simulink model "Modello_Cella_Peltier"  (R2025b)
settings: Solver=ode45  StartTime=0.0  StopTime=6600  FixedStep=0.1  MaxStep=0.5  RelTol=1e-3
libraries: slpidlib x1, simulink x1
settings Model: VariantFading=off  Creator=Lorenzo Raspaolo  LastModifiedBy=Lorenzo Raspaolo
settings SolverCC: ZeroCrossAlgorithm=Adaptive

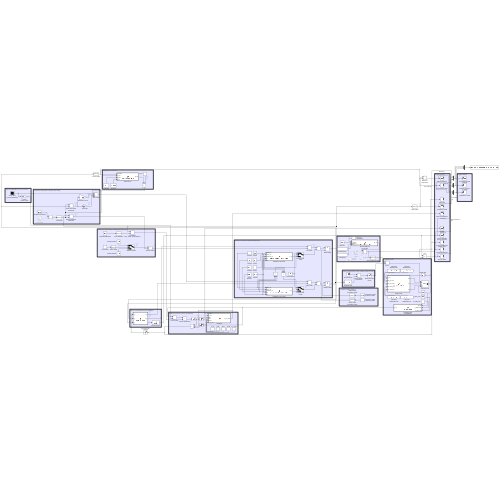
[thumbnail: Simulink's stored preview of the top-level diagram]
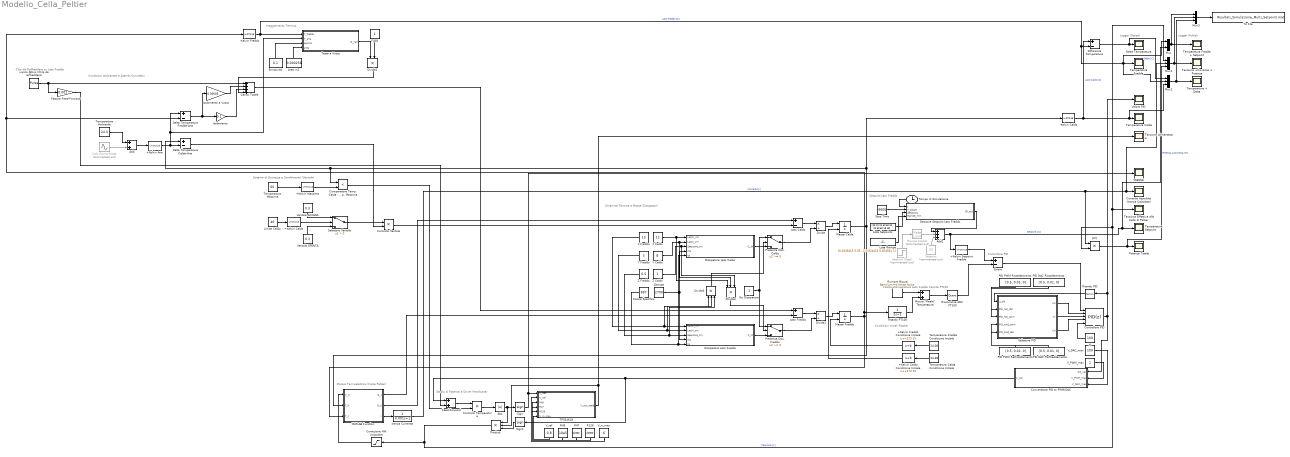
== system Modello_Cella_Peltier ==
  note: Logger Multipli
  note: Condizioni Iniziali Piastre
  note: Sistema di Sicurezza e Smaltimento (Ventola)
  note: Condizioni Ambientali e Scambi Convettivi
  note: Irraggiamento Termico
  note: Dinamica Termica e Masse (Dissipatori)
  note: Motore Termoelettrico (Fisica Peltier)
  note: Stadio di Potenza e Driver (Hardware)
  note: Controllore PID
  note: Logger (Scope)
  note: Calcolo Temperatura Lato Freddo tramite PT100
  note: Setpoint Lato Freddo
  note: Chip da Raffreddare su Lato Freddo
  +Kelvin Aria : Bias  Bias=273.15  SaturateOnIntegerOverflow=off
  +Kelvin Caldo : Bias  Bias=273.15  SaturateOnIntegerOverflow=off
  +Kelvin Caldo Condizione Iniziale : Bias  Bias=+273.15  SaturateOnIntegerOverflow=off
  +Kelvin Freddo Condizione Iniziale : Bias  Bias=+273.15  SaturateOnIntegerOverflow=off
  +Kelvin Massima : Bias  Bias=273.15  SaturateOnIntegerOverflow=off
  +Kelvin Setpoint Freddo : Bias  Bias=273.15  SaturateOnIntegerOverflow=off
  -Kelvin Caldo : Bias  Bias=-273.15  SaturateOnIntegerOverflow=off
  -Kelvin Freddo : Bias  Bias=-273.15  SaturateOnIntegerOverflow=off
  Abs : Abs  SaturateOnIntegerOverflow=off
  Add : Sum
  Add1 : Sum  Inputs=+++
  Area m2 : Constant  Value=0.000256
  Calore Specifico : Constant  Value=897
  Carico Attivo (Chip da raffreddare) : DiscretePulseGenerator  PulseType=Time based  Amplitude=0  Period=36000  PulseWidth=80  PhaseDelay=3600
  Carico Totale : Sum  Inputs=++++
  Ciclo Giorno-Notte : Sin  Commented=on  Bias=25  Frequency=2*pi/36000  SampleTime=0
  Comparatore Temp. Calda - Temp. Massima : RelationalOperator  Operator=<  OutDataTypeStr=boolean  RndMeth=Simplest  InputSameDT=off
  Controllo Temperatura : Product
  Controllo Ventola : Product
  Controllore PID : slpidlib/PID Controller  Controller=PID  Form=Parallel  TimeDomain=Discrete-time  UseExternalTs=off  SampleTime=1  IntegratorMethod=Forward Euler  FilterMethod=Forward Euler  ControllerParametersSource=external  P=1  I=0.7  UseKiTs=off  D=0  UseExternalDerivativeSource=off  N=100  UseFilter=on  TunerSelectOption=Transfer Function Based (PID Tuner App)  InitialConditionSource=internal  InitialConditionForIntegrator=0  InitialConditionForFilter=0  DifferentiatorICPrevScaledInput=0  ExternalReset=none  TrackingMode=off  Kt=1  LimitOutput=on  SatLimitsSource=internal  UpperSaturationLimit=100  LowerSaturationLimit=0  LinearizeAsGain=on  AntiWindupMode=clamping  Kb=1  LimitIntegrator=off  UpperIntegratorSaturationLimit=inf  LowerIntegratorSaturationLimit=-inf  POutMin=[]  POutMax=[]  IOutMin=[]  IOutMax=[]  DOutMin=[]  DOutMax=[]  NOutMin=[]  NOutMax=[]  SumOutMin=[]  SumOutMax=[]  SaturationOutMin=[]  SaturationOutMax=[]  PParamMin=[]  PParamMax=[]  IParamMin=[]  IParamMax=[]  DParamMin=[]  DParamMax=[]  NParamMin=[]  NParamMax=[]  KbParamMin=[]  KbParamMax=[]  KtParamMin=[]  KtParamMax=[]  KbOutMin=[]  KbOutMax=[]  KtOutMin=[]  KtOutMax=[]  IntegratorOutMin=[]  IntegratorOutMax=[]  FilterOutMin=[]  FilterOutMax=[]  SumI1OutMin=[]  SumI1OutMax=[]  SumI2OutMin=[]  SumI2OutMax=[]  SumI3OutMin=[]  SumI3OutMax=[]  SumI4OutMin=[]  SumI4OutMax=[]  SumDOutMin=[]  SumDOutMax=[]  DifferentiatorOutMin=[]  DifferentiatorOutMax=[]  FilterDiffOutCoefMin=[]  FilterDiffOutCoefMax=[]  ReciprocalOutMin=[]  ReciprocalOutMax=[]  SumDenOutMin=[]  SumDenOutMax=[]  SumNumOutMin=[]  SumNumOutMax=[]  DivideOutMin=[]  DivideOutMax=[]  UdiffTsProdOutMin=[]  UdiffTsProdOutMax=[]  NTsProdOutMin=[]  NTsProdOutMax=[]  UintegralTsProdOutMin=[]  UintegralTsProdOutMax=[]  UngainTsProdOutMin=[]  UngainTsProdOutMax=[]  ClampingZeroOutDataTypeStr=Inherit: Inherit via back propagation  ClampingZeroOutMin=[]  ClampingZeroOutMax=[]  FilterDenConstantOutDataTypeStr=Inherit: Inherit via back propagation  FilterDenConstantOutMin=[]  FilterDenConstantOutMax=[]  PCopyOutDataTypeStr=Inherit: Inherit via back propagation  PCopyOutMin=[]  PCopyOutMax=[]  NCopyOutDataTypeStr=Inherit: Inherit via back propagation  NCopyOutMin=[]  NCopyOutMax=[]  IntegratorContinuousStateAttributes=''  IntegratorStateMustResolveToSignalObject=off  IntegratorRTWStateStorageClass=Auto  FilterContinuousStateAttributes=''  FilterStateMustResolveToSignalObject=off  FilterRTWStateStorageClass=Auto  ParallelPVariant=ExternalParameters  IdealPVariant=Disabled  IVariant=ExternalParameters  DVariant=ExternalParameters  IntegratorVariant=Discrete  SatVariant=Enabled  AWVariant=DiscClampingParallel  PCopyVariant=Disabled  TRVariant=Disabled  FdbkBlocksVariant=Forward  IdealPFdbkVariant=Disabled  SatFdbkVariant=Disabled  DerivativeFilterVariant=ForwardEulerFilter  NVariant=ExternalParameters  NCopyVariant=Disabled  FilterICVariant=InternalICsFilter  IntegratorICVariant=InternalICs  ExternalResetVariant=Disabled  TRSumVariant=Passthrough  SumFdbkVariant=Disabled  SumVariant=Sum_PID  TsampFilterVariant=InternalTs  TsampNgainVariant=Passthrough  TsampIntegralVariant=Disabled_SignalSpec  ExternalSaturationOutDataTypeStr=Inherit: Same as second input  DerivativeSourceVariant=ErrorSignal  PreIntVariant=InternalPreInt
  Convertitore PID to PWM/DAC : MATLAB Function  TreatAsAtomicUnit=on
  Corrente Assorbita (Inerzia Calcolata) : Scope
      settings: ActiveDisplayYMinimum=-0.14205533461473169  ActiveDisplayYMaximum=1.2782549500001226  DataLoggingVariableName=ScopeData8
  Correzione HW Unipolare : Saturate  UpperLimit=6  LowerLimit=0
  Decisore Setpoint Lato Freddo : MATLAB Function  TreatAsAtomicUnit=on
  Delta Temperatura : Scope
      settings: ActiveDisplayYMinimum=-1  ActiveDisplayYMaximum=1  DataLoggingVariableName=ScopeData3
  Delta Temperatura Fredda-Aria : Sum  Inputs=+-
  Delta Temperatura Calda-Aria : Sum  Inputs=+-
  Densità : Constant  Value=2700
  Differenza Temperature : Sum  Inputs=+-
  Dissipatore Lato Caldo : MATLAB Function  TreatAsAtomicUnit=on
  Dissipatore Lato Freddo : MATLAB Function  TreatAsAtomicUnit=on
  Divide : Product  Inputs=*/
  Divide1 : Product  Inputs=*/
  Divide2 : Product  Inputs=**
  Divide3 : Product  Inputs=***
  Divide4 : Product  Inputs=***
  Emissività : Constant  Value=0.1
  Errore : Sum  Inputs=+-
  FLAG : Constant
  Fattore Feed-Forward : Gain  Gain=0.001
  Feed-Forward : Sum
  Inerzia Corrente : TransferFcn  Denominator=[0.001, 1]
  Isolamento : Gain  Gain=0.1
  Isolamento a Vuoto : Gain  Gain=0.00005
  Lato Caldo : Sum  Inputs=+-
  Lato Freddo : Sum  Inputs=+-
  Limite Caldo : Constant  Value=40
  Lista Rampe : Constant  Value=[0.0349415 0.0350877 0.298099 0.298246 0.429678 0.429825 0.692836 0.692982 0.824415 0.824561 1]
  Lista Setpoints : Constant  Value=[25 22 22 60 60 20 20 60 60 18 18]
  MATLAB Function : MATLAB Function  TreatAsAtomicUnit=on
  Massa Calda : Integrator  InitialConditionSource=external  InitialCondition=298.15
  Massa Fredda : Integrator  InitialConditionSource=external  InitialCondition=298.15
  "Misura \"Reale\" Temperatura" : Sum
  Mux : Mux  Inputs=2
  Mux1 : Mux  Inputs=3
  Mux2 : Mux  Inputs=3
  Mux3 : Mux  Inputs=3
  N : Constant  Value=100
  No Dissipatore : Constant
  PID DAC Raffreddamento : Constant  Value=[0.5, 0.01, 0]
  PID DAC Riscaldamento : Constant  Value=[0.5, 0.01, 0]
  PID PWM Raffreddamento : Constant  Value=[0.5, 0.01, 0]
  PID PWM Riscaldamento : Constant  Value=[0.5, 0.01, 0]
  Potenza Totale : Scope
      settings: DataLoggingVariableName=ScopeData13
  Presenza Diss. Caldo : Switch  SaturateOnIntegerOverflow=off  InputSameDT=off
  Presenza Diss. Freddo : Switch  SaturateOnIntegerOverflow=off  InputSameDT=off
  Product : Product  Inputs=3
  R126 : Constant  Value=22000
  R45 : Constant  Value=10e5
  R47 : Constant  Value=24300
  Rampa Freddo : RateLimiter  Commented=on  RisingSlewLimit=1/60  FallingSlewLimit=-1/60  SampleTimeMode=inherited
  Risoluzione ADC PT100 : Quantizer  QuantizationInterval=0.05
  Ritardo PID : Memory
  Ritardo PT100 : TransferFcn  Denominator=[2 1]
  Rumore Misura : simulink/Sources/Band-Limited White Noise  Cov=[0.001]  Ts=0.1  seed=[23341]
  Selettore PID : MATLAB Function  TreatAsAtomicUnit=on
  Selettore Ventola : Switch  Criteria=u2 > Threshold  SaturateOnIntegerOverflow=off  InputSameDT=off
  Setpoint : Constant  Commented=on  Value=20
  Setpoint (Step) : Step  Commented=on  Time=18000  Before=25  After=35  SampleTime=0
  Sign : Signum
  Sign1 : Signum
  Stop Time : Constant  Value=6600
  TPS54618 : MATLAB Function  TreatAsAtomicUnit=on
  Temperatura Ambiente : Constant  Value=24.0
  Temperatura Calda : Scope
      settings: ActiveDisplayYMinimum=24.820001034825616  ActiveDisplayYMaximum=25.473742804218269  DataLoggingMaxPoints=100000
  Temperatura Calda Condizione Iniziale : Constant  Value=24.38
  Temperatura Fredda : Scope
      settings: ActiveDisplayYMinimum=12.498230635091431  ActiveDisplayYMaximum=37.510882671126524  DataLoggingMaxPoints=100000
  Temperatura Fredda + Setpoint : Scope
      settings: ActiveDisplayYMinimum=11.365475528684039  ActiveDisplayYMaximum=65.403836052368447  DataLoggingVariableName=ScopeData11
  Temperatura Fredda Condizione Iniziale : Constant  Value=24.08
  Temperatura Massima : Constant  Value=60
  Temperatura Setpoint : Scope
      settings: ActiveDisplayYMinimum=12.5  ActiveDisplayYMaximum=37.5  DataLoggingVariableName=ScopeData10
  Temperature + Delta : Scope
      settings: ActiveDisplayYMinimum=-3.0766667374527747  ActiveDisplayYMaximum=30.690000637075094  DataLoggingVariableName=ScopeData14
  Tempo di Simulazione : Clock
  Tensione +Corrente + Potenza : Scope
      settings: ActiveDisplayYMinimum=-0.099999999999999978  ActiveDisplayYMaximum=0.9  DataLoggingVariableName=ScopeData12
  Tensione Alimentatore : Scope
      settings: ActiveDisplayYMinimum=0.9360873097501603  ActiveDisplayYMaximum=1.0071022514812031  DataLoggingVariableName=ScopeData5
  Tensione Effettiva alla Cella di Peltier : Scope
      settings: ActiveDisplayYMinimum=-3.9749734687625553  ActiveDisplayYMaximum=2.3792612188630025  DataLoggingVariableName=ScopeData9
  Testa a Vuoto : MATLAB Function  TreatAsAtomicUnit=on
  To File : ToFile  Filename=Risultati_Simulazione_Multi_Setpoint.mat  SaveFormat=Timeseries
  VSENSE : Scope
      settings: ActiveDisplayYMinimum=-1  ActiveDisplayYMaximum=1  DataLoggingVariableName=ScopeData7
  V_DAC_max : Constant  Value=100
  V_PWM_max : Constant
  V_in_max : Constant  Value=6
  V_ref : Constant  Value=0.8
  Valore PID : Scope
      settings: ActiveDisplayYMinimum=-175.48303125000382  ActiveDisplayYMaximum=88.847281250034527  DataLoggingMaxPoints=100000  DataLoggingVariableName=ScopeData4
  Ventola ACCESA : Constant  Value=0.3
  Ventola SPENTA : Constant  Value=0.3
  X Caldo : Constant  Value=12
  X Freddo : Constant  Value=13
  Y Caldo : Constant  Value=8
  Y Freddo : Constant  Value=3
  Z Caldo : Constant
  Z Freddo : Constant  Value=0.5
  "[W]" : Product
  wires:
  Isolamento/1 -> Carico Totale/3
  Isolamento a Vuoto/1 -> Carico Totale/2
  Setpoint/1 -> Add1/3
  Y Freddo/1 -> Dissipatore Lato Freddo/2(LatoY_cm), Divide3/2
  Carico Attivo (Chip da raffreddare)/1 -> Carico Totale/1, Fattore Feed-Forward/1
  Divide/1 -> Massa Calda/1
  +Kelvin Aria/1 -> Testa a Vuoto/2(T_aria), Delta Temperatura Fredda-Aria/1, Delta Temperatura Calda-Aria/2
  Delta Temperatura Fredda-Aria/1 -> Isolamento a Vuoto/1, Isolamento/1
  Feed-Forward/1 -> Controllo Temperatura/1
  Z Caldo/1 -> Dissipatore Lato Caldo/3(Spessore_cm), Divide4/3
  Y Caldo/1 -> Dissipatore Lato Caldo/2(LatoY_cm), Divide4/2
  Densità/1 -> Dissipatore Lato Caldo/4(rho), Dissipatore Lato Freddo/4(rho)
  Calore Specifico/1 -> Dissipatore Lato Freddo/5(cp), Dissipatore Lato Caldo/5(cp)
  "Misura \"Reale\" Temperatura"/1 -> Risoluzione ADC PT100/1
  X Caldo/1 -> Dissipatore Lato Caldo/1(LatoX_cm), Divide4/1
  -Kelvin Freddo/1 -> Mux2/2, Temperatura Fredda/1, Mux/1, Differenza Temperature/2, Testa a Vuoto/1(T_fredda)  "Lato Freddo [C]"
  Selettore Ventola/1 -> Controllo Ventola/1
  Massa Fredda/1 -> Ritardo PT100/1, -Kelvin Freddo/1, Delta Temperatura Fredda-Aria/2, MATLAB Function/3(T_c)
  Z Freddo/1 -> Dissipatore Lato Freddo/3(Spessore_cm), Divide3/3
  X Freddo/1 -> Dissipatore Lato Freddo/1(LatoX_cm), Divide3/1
  Divide1/1 -> Massa Fredda/1
  Controllore PID/1 -> Valore PID/1, Ritardo PID/1, Convertitore PID to PWM/DAC/1(pid_val)
  Massa Calda/1 -> -Kelvin Caldo/1, Comparatore Temp. Calda - Temp. Massima/1, Delta Temperatura Calda-Aria/1, MATLAB Function/2(T_h)
  +Kelvin Caldo/1 -> Selettore Ventola/2
  Emissività/1 -> Testa a Vuoto/3(epsilon)
  Errore/1 -> Controllore PID/1
  N/1 -> Controllore PID/5
  +Kelvin Setpoint Freddo/1 -> Errore/1
  Rumore Misura/1 -> "Misura \"Reale\" Temperatura"/1
  Ritardo PT100/1 -> "Misura \"Reale\" Temperatura"/2
  Ventola ACCESA/1 -> Selettore Ventola/1
  MATLAB Function/3(I) -> Inerzia Corrente/1
  Sign/1 -> TPS54618/1(V_dac), VSENSE/1
  Ventola SPENTA/1 -> Selettore Ventola/3
  Limite Caldo/1 -> +Kelvin Caldo/1
  Temperatura Massima/1 -> +Kelvin Massima/1
  +Kelvin Massima/1 -> Comparatore Temp. Calda - Temp. Massima/2
  Area m2/1 -> Testa a Vuoto/4(area)
  Abs/1 -> Product/1, Sign/1
  TPS54618/1(V_out_reale) -> Product/2, Tensione Alimentatore/1
  -Kelvin Caldo/1 -> Differenza Temperature/1, Mux2/3, Temperatura Calda/1  "Lato Caldo [C]"
  Carico Totale/1 -> Lato Freddo/1
  Risoluzione ADC PT100/1 -> Errore/2
  Delta Temperatura Calda-Aria/1 -> Controllo Ventola/2
  Fattore Feed-Forward/1 -> Feed-Forward/2
  Controllo Ventola/1 -> Lato Caldo/2
  Comparatore Temp. Calda - Temp. Massima/1 -> Controllo Temperatura/2
  MATLAB Function/1(Q_c) -> Lato Freddo/2
  MATLAB Function/2(Q_h) -> Lato Caldo/1
  Inerzia Corrente/1 -> "[W]"/1, Corrente Assorbita (Inerzia Calcolata)/1, Mux1/2  "Corrente [I]"
  Lato Caldo/1 -> Divide/1
  Lato Freddo/1 -> Divide1/1
  Differenza Temperature/1 -> Mux2/1, Delta Temperatura/1  "Delta [C]"
  Testa a Vuoto/1(Q_rad) -> Divide2/1
  Divide2/1 -> Carico Totale/4
  FLAG/1 -> Divide2/2
  Temperatura Fredda Condizione Iniziale/1 -> +Kelvin Freddo Condizione Iniziale/1
  Temperatura Calda Condizione Iniziale/1 -> +Kelvin Caldo Condizione Iniziale/1
  +Kelvin Freddo Condizione Iniziale/1 -> Massa Fredda/2
  +Kelvin Caldo Condizione Iniziale/1 -> Massa Calda/2
  Controllo Temperatura/1 -> Abs/1
  Product/1 -> "[W]"/2, Mux1/1, Tensione Effettiva alla Cella di Peltier/1, Correzione HW Unipolare/1  "Tensione [V]"
  Dissipatore Lato Freddo/1(C_tc) -> Presenza Diss. Freddo/3
  Dissipatore Lato Caldo/1(C_th) -> Presenza Diss. Caldo/3
  No Dissipatore/1 -> Presenza Diss. Freddo/1, Presenza Diss. Caldo/1
  Presenza Diss. Caldo/1 -> Divide/2
  Presenza Diss. Freddo/1 -> Divide1/2
  Divide4/1 -> Presenza Diss. Freddo/2
  Divide3/1 -> Presenza Diss. Caldo/2
  V_PWM_max/1 -> Convertitore PID to PWM/DAC/2(V_PWM_max)
  V_DAC_max/1 -> Convertitore PID to PWM/DAC/3(V_DAC_max)
  Convertitore PID to PWM/DAC/1(V_out) -> Feed-Forward/1, Sign1/1
  Sign1/1 -> Product/3
  Add1/1 -> Temperatura Setpoint/1, Mux/2, +Kelvin Setpoint Freddo/1  "Setpoint [C]"
  Setpoint (Step)/1 -> Rampa Freddo/1
  Add/1 -> +Kelvin Aria/1
  Ciclo Giorno-Notte/1 -> Add/2
  Temperatura Ambiente/1 -> Add/1
  Tempo di Simulazione/1 -> Decisore Setpoint Lato Freddo/1(t)
  Rampa Freddo/1 -> Add1/2
  Decisore Setpoint Lato Freddo/1(SP_out) -> Add1/1
  Lista Setpoints/1 -> Decisore Setpoint Lato Freddo/3(Setpoints)
  Lista Rampe/1 -> Decisore Setpoint Lato Freddo/4(Rampe_min)
  Stop Time/1 -> Decisore Setpoint Lato Freddo/2(T_totale)
  Mux/1 -> Mux3/1, Temperatura Fredda + Setpoint/1
  Mux1/1 -> Mux3/2, Tensione +Corrente + Potenza/1
  "[W]"/1 -> Mux1/3, Potenza Totale/1  "Potenza Assorbita [W]"
  Mux2/1 -> Mux3/3, Temperature + Delta/1
  V_ref/1 -> TPS54618/6(V_in_max)
  R45/1 -> TPS54618/5(R126)
  R47/1 -> TPS54618/4(R47)
  R126/1 -> TPS54618/3(R45)
  V_in_max/1 -> TPS54618/2(V_ref)
  Selettore PID/2(Ki) -> Controllore PID/3
  Selettore PID/1(Kp) -> Controllore PID/2
  Selettore PID/3(Kd) -> Controllore PID/4
  Ritardo PID/1 -> Selettore PID/1(u_pid)
  PID PWM Raffreddamento/1 -> Selettore PID/4(PID_cold_pwm)
  PID DAC Raffreddamento/1 -> Selettore PID/5(PID_cold_dac)
  PID PWM Riscaldamento/1 -> Selettore PID/3(PID_hot_pwm)
  PID DAC Riscaldamento/1 -> Selettore PID/2(PID_hot_dac)
  Mux3/1 -> To File/1
  Correzione HW Unipolare/1 -> MATLAB Function/1(V_in)

== matlab function Modello_Cella_Peltier/Testa a Vuoto ==
  data: T_fredda input; T_aria input; Q_rad output; epsilon input; area input
function Q_rad = Calcolo_Irraggiamento(T_fredda, T_aria, epsilon, area)
    % Costante di Stefan-Boltzmann (W/m^2*K^4)
    sigma = 5.67e-8;
    
    % Calcolo del calore per irraggiamento
    Q_rad = epsilon * sigma * area * (T_aria^4 - T_fredda^4);
end

== matlab function Modello_Cella_Peltier/MATLAB Function ==
  data: V_in input; Q_c output; T_h input; T_c input; Q_h output; I output
function [Q_c, Q_h, I] = Cella_di_Peltier(V_in, T_h, T_c)
    % peltier_core: Calcola le potenze termiche e la corrente di una cella Peltier
    % V_in : Tensione applicata (Volt)
    % T_h  : Temperatura lato caldo (Kelvin)
    % T_c  : Temperatura lato freddo (Kelvin)
    
    % 1. Calcolo parametri termici base
    T_med = (T_h + T_c) / 2;
    dT = T_h - T_c;

    % 2. Polinomi del Tellururo di Bismuto (scalati per RC3-2.5 + Res. Parassita)
    alfa = 0.515 * (0.0133450 - 0.0000537574*T_med + 0.000000742731*T_med^2 - 0.00000000127141*T_med^3);
    R = 1.51 * (2.08317 - 0.0198763*T_med + 0.0000853832*T_med^2 - 0.0000000903143*T_med^3);
    K = 0.185 * (0.476218 - 0.00000389821*T_med - 0.00000864864*T_med^2 + 0.0000000220869*T_med^3);

    % 3. Calcolo Corrente Effettiva (Legge di Ohm modificata da Seebeck)
    I = (V_in - (alfa * dT)) / R;

    % 4. Calcolo Potenze Termiche (Watt)
    % Q_c = Calore estratto dal lato freddo (se positivo, raffredda)
    Q_c = (alfa * I * T_c) - (0.5 * I^2 * R) - (K * dT);
    
    % Q_h = Calore espulso dal lato caldo (verso il dissipatore)
    Q_h = (alfa * I * T_h) + (0.5 * I^2 * R) - (K * dT);

    % Corrente assorbita positiva
    I = abs(I);
end

== matlab function Modello_Cella_Peltier/Convertitore PID to PWM//DAC ==
  data: pid_val input; V_out output; V_PWM_max input; V_DAC_max input
function V_out = controllo_ibrido(pid_val, V_PWM_max, V_DAC_max)
    % Calcoliamo il valore assoluto e memorizziamo il segno (+ o -)
    u_abs = abs(pid_val);
    segno = sign(pid_val);
    
    % Inizializziamo la tensione
    v_eff = 0;
    
    if u_abs <= 100
        % --- ZONA PWM (0 - 100) ---
        % Calcola il Duty Cycle (da 0.0 a 1.0)
        duty = u_abs / 100;
        v_eff = duty * V_PWM_max;
        
    elseif u_abs <= 200
        % --- ZONA DAC (100 - 200) ---
        % Calcola la percentuale di intervento del DAC (da 0.0 a 1.0)
        k = (u_abs - 100) / 100;
        v_eff = V_PWM_max + (k * (V_DAC_max - V_PWM_max));
        
    else
        % --- SATURAZIONE DI SICUREZZA ---
        % Se il PID impazzisce oltre 200, limitiamo al massimo
        v_eff = V_DAC_max;
    end
    
    % Riapplichiamo il segno per dire al ponte H da che lato spingere
    V_out = v_eff * segno;
end

== matlab function Modello_Cella_Peltier/Dissipatore Lato Freddo ==
  data: LatoX_cm input; C_tc output; LatoY_cm input; Spessore_cm input; rho input; cp input
function C_tc = calcola_capacita_termica_freddo(LatoX_cm, LatoY_cm, Spessore_cm, rho, cp)
    % Converte i cm in metri per il calcolo del volume
    volume_m3 = (LatoX_cm / 100) * (LatoY_cm / 100) * (Spessore_cm / 100);
    
    % Calcola la massa in kg (Volume * Densità)
    massa_kg = volume_m3 * rho;
    
    % Calcola la Capacità Termica in J/K (Massa * Calore Specifico)
    C_tc = massa_kg * cp;
end

== matlab function Modello_Cella_Peltier/Dissipatore Lato Caldo ==
  data: LatoX_cm input; C_th output; LatoY_cm input; Spessore_cm input; rho input; cp input
function C_th = calcola_capacita_termica_caldo(LatoX_cm, LatoY_cm, Spessore_cm, rho, cp)
    % Converte i cm in metri per il calcolo del volume
    volume_m3 = (LatoX_cm / 100) * (LatoY_cm / 100) * (Spessore_cm / 100);
    
    % Calcola la massa in kg (Volume * Densità)
    massa_kg = volume_m3 * rho;
    
    % Calcola la Capacità Termica in J/K (Massa * Calore Specifico)
    C_th = massa_kg * cp;
end

== matlab function Modello_Cella_Peltier/Decisore Setpoint Lato Freddo ==
  data: t input; T_totale input; SP_out output; Setpoints input; Rampe_min input
function SP_out = profilatore_termico_fasi(t, T_totale, Setpoints, Rampe_min)
    % t: tempo attuale dal blocco Clock
    % Setpoints: es. [25, 15, -10]
    % Rampe_min: es. [1, 2] (gradi al minuto)
    % T_totale: tempo totale della simulazione in secondi (es. 36000)

    N_fasi = length(Setpoints);
    % Calcoliamo la durata di ogni "fetta" di simulazione
    T_fase = T_totale / N_fasi; 
    
    % Capiamo in quale fase ci troviamo (1, 2, o 3...)
    fase_attuale = floor(t / T_fase) + 1;
    
    % Sicurezza: se il tempo arriva esattamente alla fine, restiamo nell'ultima fase
    if fase_attuale > N_fasi
        fase_attuale = N_fasi;
    end
    
    % --- Calcolo del Setpoint ---
    if fase_attuale == 1
        % Fase 1: Manteniamo il setpoint di partenza per farlo andare a regime
        SP_out = Setpoints(1);
    else
        % Fasi successive: Iniziamo la rampa
        t_inizio_fase = (fase_attuale - 1) * T_fase;
        
        SP_iniziale = Setpoints(fase_attuale - 1);
        SP_bersaglio = Setpoints(fase_attuale);
        
        rate_sec = Rampe_min(fase_attuale - 1) / 60;
        segno = sign(SP_bersaglio - SP_iniziale);
        
        % Quanto tempo è passato dall'inizio di QUESTA fase?
        dt = t - t_inizio_fase;
        
        % Calcoliamo la nuova temperatura
        SP_calcolato = SP_iniziale + (segno * rate_sec * dt);
        
        % SATURAZIONE: Se la rampa ha raggiunto il bersaglio, fermiamola!
        % Così il sistema avrà il resto del tempo della fase per stabilizzarsi (Soak Time)
        if segno == 1 && SP_calcolato > SP_bersaglio
            SP_out = SP_bersaglio;
        elseif segno == -1 && SP_calcolato < SP_bersaglio
            SP_out = SP_bersaglio;
        elseif rate_sec == 0
            SP_out = SP_bersaglio;
        else
            SP_out = SP_calcolato; % La rampa è ancora in corso
        end
    end
end

== matlab function Modello_Cella_Peltier/TPS54618 ==
  data: V_dac input; V_out_reale output; V_ref input; R45 input; R47 input; R126 input; V_in_max input
function V_out_reale = TPS54618_Hardware(V_dac, V_ref, R45, R47, R126, V_in_max)
    % V_dac: Segnale di controllo dal PID/Generatore PWM
    % V_ref: Tensione di riferimento interna del TPS54618 (es. 0.8V)
    % R45: Resistenza Top del partitore (es. 100000 ohm)
    % R47: Resistenza Bottom verso GND (es. 24300 ohm)
    % R126: Resistenza di iniezione dal DAC (es. 22000 ohm)
    % V_in_max: Tensione di alimentazione del convertitore (es. 5V)

    % Equazione di Kirchhoff del nodo VSNS
    V_calcolata = V_ref * (1 + (R45/R47) + (R45/R126)) - V_dac * (R45/R126);
    
    % Saturazione hardware (Il buck non può dare voltaggi negativi 
    % e non può superare la tensione di alimentazione)
    if V_calcolata > V_in_max
        V_out_reale = V_in_max;
    elseif V_calcolata < 0
        V_out_reale = 0;
    else
        V_out_reale = V_calcolata;
    end
end

== matlab function Modello_Cella_Peltier/Selettore PID ==
  data: u_pid input; Kp output; Ki output; Kd output; PID_hot_dac input; PID_hot_pwm input; PID_cold_pwm input; PID_cold_dac input
function [Kp, Ki, Kd] = selettore_guadagni(u_pid, PID_hot_dac, PID_hot_pwm, PID_cold_pwm, PID_cold_dac)
    % u_pid: valore del PID ritardato dal blocco Memory
    % PID_... : Vettori in ingresso con formato [P, I, D]

    % --- LOGICA DI SELEZIONE ---
    if u_pid >= 100
        % 1. Riscaldamento DAC
        Kp = PID_hot_dac(1);
        Ki = PID_hot_dac(2);
        Kd = PID_hot_dac(3);
        
    elseif u_pid >= 0 && u_pid < 100
        % 2. Riscaldamento PWM
        Kp = PID_hot_pwm(1);
        Ki = PID_hot_pwm(2);
        Kd = PID_hot_pwm(3);
        
    elseif u_pid < 0 && u_pid >= -100
        % 3. Raffreddamento PWM
        Kp = PID_cold_pwm(1);
        Ki = PID_cold_pwm(2);
        Kd = PID_cold_pwm(3);
        
    else % u_pid < -100
        % 4. Raffreddamento DAC
        Kp = PID_cold_dac(1);
        Ki = PID_cold_dac(2);
        Kd = PID_cold_dac(3);
    end
end
